simulink model "FullModel_v3_noYaw"  (R2018a)
settings: Solver=FixedStepAuto  StartTime=0.0  StopTime=Inf  FixedStep=0.01  RelTol=1e-3
undefined symbols (not defined in the file or in its folder): none, videoinput, XZini
libraries: simulink x2, imaqlib x1
settings Model: SimulationMode=accelerator  Creator=Alex  LastModifiedBy=Alex
settings OptimizationCC: EfficientMapNaN2IntZero=off
settings HardwareCC: TargetBitPerLong=64  TargetBitPerPointer=64  TargetBitPerSizeT=64  TargetBitPerPtrDiffT=64  TargetLongLongMode=on  TargetIntDivRoundTo=Zero  TargetEndianess=LittleEndian  TargetWordSize=64  TargetHWDeviceType=MATLAB Host  ProdEqTarget=off
settings CodeAppCC: MaxIdLength=128
settings GRTTargetCC: TargetLangStandard=C89/C90 (ANSI)  CombineOutputUpdateFcns=off  GRTInterface=on

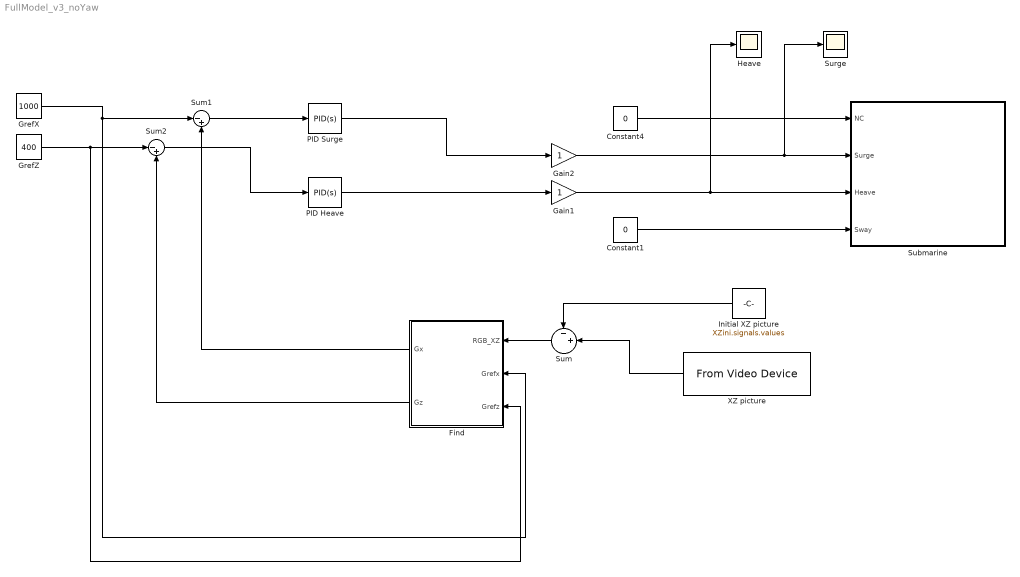
== system FullModel_v3_noYaw ==
  Constant1 : Constant  Value=0
  Constant4 : Constant  Value=0
  Find : MATLAB Function  TreatAsAtomicUnit=on
  Gain1 : Gain
  Gain2 : Gain
  GrefX : Constant  Value=1000
  "GrefZ " : Constant  Value=400
  Heave : Scope
  Initial XZ picture : Constant  Value=XZini.signals.values
  PID Heave : simulink/Continuous/PID Controller  Controller=PID  TimeDomain=Continuous-time  SampleTime=-1  IntegratorMethod=Forward Euler  FilterMethod=Forward Euler  Form=Parallel  UseFilter=on  ControllerParametersSource=internal  P=8  I=3  D=0  N=100  InitialConditionSource=internal  InitialConditionForIntegrator=0  InitialConditionForFilter=0  ExternalReset=none  LimitOutput=on  UpperSaturationLimit=1000  LowerSaturationLimit=-1000  LinearizeAsGain=on  AntiWindupMode=none  Kb=1  TrackingMode=off  Kt=1  PParamMin=[]  PParamMax=[]  IParamMin=[]  IParamMax=[]  DParamMin=[]  DParamMax=[]  NParamMin=[]  NParamMax=[]  KbParamMin=[]  KbParamMax=[]  KtParamMin=[]  KtParamMax=[]  POutMin=[]  POutMax=[]  IOutMin=[]  IOutMax=[]  DOutMin=[]  DOutMax=[]  NOutMin=[]  NOutMax=[]  KbOutMin=[]  KbOutMax=[]  KtOutMin=[]  KtOutMax=[]  IntegratorOutMin=[]  IntegratorOutMax=[]  FilterOutMin=[]  FilterOutMax=[]  SumOutMin=[]  SumOutMax=[]  SumI1OutMin=[]  SumI1OutMax=[]  SumI2OutMin=[]  SumI2OutMax=[]  SumI3OutMin=[]  SumI3OutMax=[]  SumDOutMin=[]  SumDOutMax=[]  SaturationOutMin=[]  SaturationOutMax=[]  IntegratorContinuousStateAttributes=''  IntegratorStateMustResolveToSignalObject=off  IntegratorRTWStateStorageClass=Auto  FilterContinuousStateAttributes=''  FilterStateMustResolveToSignalObject=off  FilterRTWStateStorageClass=Auto  DifferentiatorICPrevScaledInput=0  DifferentiatorOutMin=[]  DifferentiatorOutMax=[]  FilterDiffOutCoefMin=[]  FilterDiffOutCoefMax=[]  SumDenOutMin=[]  SumDenOutMax=[]  SumNumOutMin=[]  SumNumOutMax=[]  ReciprocalOutMin=[]  ReciprocalOutMax=[]  DivideOutMin=[]  DivideOutMax=[]  TunerSelectOption=Transfer Function Based (PID Tuner App)
  PID Surge : simulink/Continuous/PID Controller  Controller=PID  TimeDomain=Continuous-time  SampleTime=-1  IntegratorMethod=Forward Euler  FilterMethod=Forward Euler  Form=Parallel  UseFilter=on  ControllerParametersSource=internal  P=4  I=1.75  D=0  N=100  InitialConditionSource=internal  InitialConditionForIntegrator=0  InitialConditionForFilter=0  ExternalReset=none  LimitOutput=on  UpperSaturationLimit=700  LowerSaturationLimit=-700  LinearizeAsGain=on  AntiWindupMode=none  Kb=1  TrackingMode=off  Kt=1  PParamMin=[]  PParamMax=[]  IParamMin=[]  IParamMax=[]  DParamMin=[]  DParamMax=[]  NParamMin=[]  NParamMax=[]  KbParamMin=[]  KbParamMax=[]  KtParamMin=[]  KtParamMax=[]  POutMin=[]  POutMax=[]  IOutMin=[]  IOutMax=[]  DOutMin=[]  DOutMax=[]  NOutMin=[]  NOutMax=[]  KbOutMin=[]  KbOutMax=[]  KtOutMin=[]  KtOutMax=[]  IntegratorOutMin=[]  IntegratorOutMax=[]  FilterOutMin=[]  FilterOutMax=[]  SumOutMin=[]  SumOutMax=[]  SumI1OutMin=[]  SumI1OutMax=[]  SumI2OutMin=[]  SumI2OutMax=[]  SumI3OutMin=[]  SumI3OutMax=[]  SumDOutMin=[]  SumDOutMax=[]  SaturationOutMin=[]  SaturationOutMax=[]  IntegratorContinuousStateAttributes=''  IntegratorStateMustResolveToSignalObject=off  IntegratorRTWStateStorageClass=Auto  FilterContinuousStateAttributes=''  FilterStateMustResolveToSignalObject=off  FilterRTWStateStorageClass=Auto  DifferentiatorICPrevScaledInput=0  DifferentiatorOutMin=[]  DifferentiatorOutMax=[]  FilterDiffOutCoefMin=[]  FilterDiffOutCoefMax=[]  SumDenOutMin=[]  SumDenOutMax=[]  SumNumOutMin=[]  SumNumOutMax=[]  ReciprocalOutMin=[]  ReciprocalOutMax=[]  DivideOutMin=[]  DivideOutMax=[]  TunerSelectOption=Transfer Function Based (PID Tuner App)
  Submarine : Subsystem
  Sum : Sum  Inputs=-+|
  Sum1 : Sum  Inputs=|-+
  Sum2 : Sum  Inputs=|-+
  Surge : Scope
  XZ picture : imaqlib/From Video Device  DeviceMenu=macvideo 2 (USB Camera)  Device=macvideo 2 (USB Camera)  ObjConstructor=videoinput('macvideo', 2)  VideoFormatMenu=YCbCr422_1920x1080  VideoFormat=YCbCr422_1920x1080  VideoSource=default  ROIPosition=[0 0 1080 1920]  EnableHWTrigger=off  TriggerConfiguration=none/none  SampleTime=0.01  OutputPortsMode=One multidimensional signal  DataType=double  CanDoHWTrigger=no  ReturnedColorSpace=rgb  BlockHandle=6.0002  ROIWidth=1920  ROIHeight=1080  ROIColumn=0  ROIRow=0  EngXMLPath=/Applications/MATLAB_R2018a.app/toolbox/imaq/imaq/private  DevXMLPath=/Users/Alex/Documents/MATLAB/SupportPackages/R2018a/toolbox/imaq/supportpackages/genericvideo/adaptor/maci64  EngLibPath=/Applications/MATLAB_R2018a.app/toolbox/imaq/imaqblks/imaqmex/maci64  ColorSpace=rgb  BayerSensorAlignment=grbg
      settings: SourceProductName=Image Acquisition Toolbox
  wires:
  Initial XZ picture/1 -> Sum/1
  XZ picture/1 -> Sum/2
  Sum/1 -> Find/1(RGB_XZ)
  Find/1(Gx) -> Sum1/2
  GrefX/1 -> Sum1/1, Find/2(Grefx)
  "GrefZ "/1 -> Sum2/1, Find/3(Grefz)
  Find/2(Gz) -> Sum2/2
  Sum1/1 -> PID Surge/1
  Sum2/1 -> PID Heave/1
  Constant4/1 -> Submarine/1(NC)
  Gain1/1 -> Heave/1, Submarine/3(Heave)
  Gain2/1 -> Surge/1, Submarine/2(Surge)
  Constant1/1 -> Submarine/4(Sway)
  PID Surge/1 -> Gain2/1
  PID Heave/1 -> Gain1/1

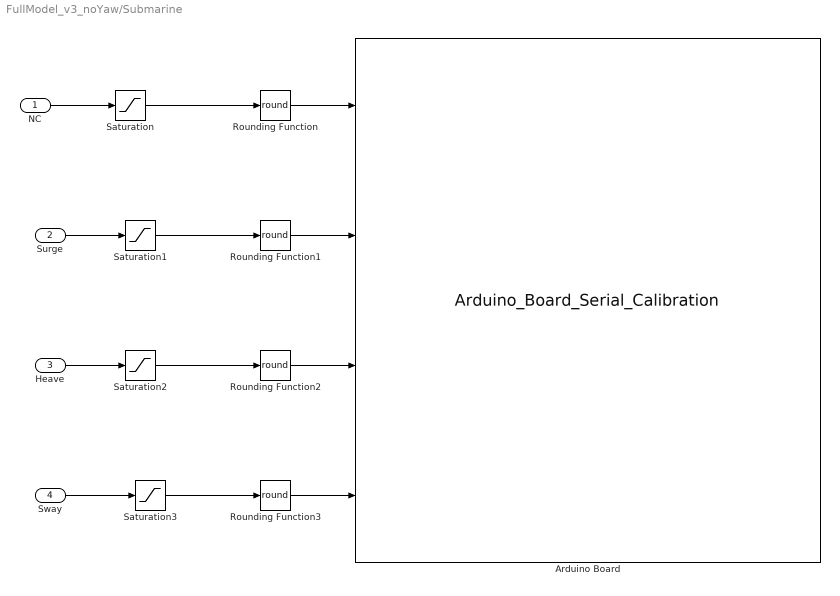
== system FullModel_v3_noYaw/Submarine ==
  NC : Inport
  Surge : Inport  Port=2
  Heave : Inport  Port=3
  Sway : Inport  Port=4
  Arduino Board : M-S-Function  FunctionName=Arduino_Board_Serial_Calibration  mask(Arduino Board){ComPort='/dev/cu.usbmodem143441', BLDC_Enable=on}
      mask prompts: ComPort "Port"; BLDC_Enable "Enable BLDC Rotor"
      mask help: Define the selected Port [e.g. 'Com4'] for the Arduino board and enable the brushless DC motor.
      mask DialogControl Container5 Prompt: Enables
      mask Display:
      | port_label('input',1,'DesiredSpeed_1')
      | port_label('input',2,'DesiredSpeed_2')
      | port_label('input',3,'DesiredSpeed_3')
      | port_label('input',4,'DesiredSpeed_4')
      | port_label('input',5,'DesiredAngle_1')
      | port_label('input',6,'DesiredAngle_2')
      | port_label('input',7,'DesiredAngle_3')
      | port_label('input',8,'DesiredAngle_4')
      | port_label('input',9,'DesiredLinear')
      | port_label('output',1,'Speed 1')
      | port_label('output',2,'Speed 2')
      | port_label('output',3,'Speed 3')
      | port_label('output',4,'Speed 4')
      | port_label('output',5,'Angle 5')
      | port_label('output',6,'Angle 6')
      | port_label('output',7,'Angle 7')
      | port_label('output',8,'Angle 8')
      | port_label('output',9,'Linear 9')
      | fprintf('Arduino\n Board');
  Rounding Function{,1..3} (4 alike) : Rounding  Operator=round
  Saturation{,1..3} (4 alike) : Saturate  UpperLimit=1000  LowerLimit=-1000
  wires:
  NC/1 -> Saturation/1
  Rounding Function/1 -> Arduino Board/1
  Surge/1 -> Saturation1/1
  Rounding Function1/1 -> Arduino Board/2
  Heave/1 -> Saturation2/1
  Rounding Function2/1 -> Arduino Board/3
  Sway/1 -> Saturation3/1
  Rounding Function3/1 -> Arduino Board/4
  Saturation3/1 -> Rounding Function3/1
  Saturation2/1 -> Rounding Function2/1
  Saturation1/1 -> Rounding Function1/1
  Saturation/1 -> Rounding Function/1

== matlab function FullModel_v3_noYaw/Find ==
  data: Gx output; Gz output; RGB_XZ input; Grefx input; Grefz input
function [Gx, Gz]  = fcn(RGB_XZ,Grefx,Grefz)
    coder.extrinsic('image')
    
    % Parameters
    Acrit     = 0.6; % Blue LED detection criteria
    
    % Keep red signal from RGB
    A = RGB_XZ(:,:,3);

    % Find Blue LED in picture
    [Iz, Ix] = find(A>Acrit);
    Iz       = 1080 - Iz;
    
    % Compute Submarine's Center of Gravity
    Gx = mean(Ix) ;
    Gz = mean(Iz);

    
    % Check plots
     %figure(1)
     %plot(Gx,Gz,'r+','MarkerSize',10); axis([0 1920 0 1080]); grid on; hold on;
     %plot(Grefx,Grefz,'go','MarkerSize',20,'LineWidth',4);
     %hold off;

end
